simulink model "iqrdrls_simulink"  (R2012b)
settings: Solver=FixedStepDiscrete  SolverMode=SingleTasking  StartTime=0.0  StopTime=2450  RelTol=1e-3
libraries: dspsigops x5
settings Model: MinMaxOverflowLogging=MinMaxAndOverflow  FPTRunName=NoOverride  Creator=andreas  LastModifiedBy=andreas
settings DataIOCC: InspectSignalLogs=on
settings OptimizationCC: InlineParams=on  SimCompilerOptimization=On
settings DebuggingCC: SignalRangeChecking=warning  ParameterDowncastMsg=warning  ParameterOverflowMsg=warning  StrictBusMsg=ErrorOnBusTreatedAsVector  LoggingUnavailableSignals=none
settings HardwareCC: ProdHWDeviceType=Generic->Unspecified (assume 32-bit Generic)  TargetBitPerLong=64  TargetBitPerPointer=64  TargetIntDivRoundTo=Zero  TargetEndianess=LittleEndian  TargetWordSize=64  TargetHWDeviceType=MATLAB Host  ProdEqTarget=off
settings ModelReferenceCC: EnableParallelModelReferenceBuilds=on

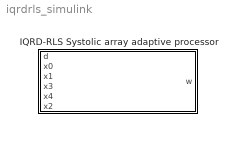
== system iqrdrls_simulink ==
  IQRD-RLS Systolic array adaptive processor : Subsystem

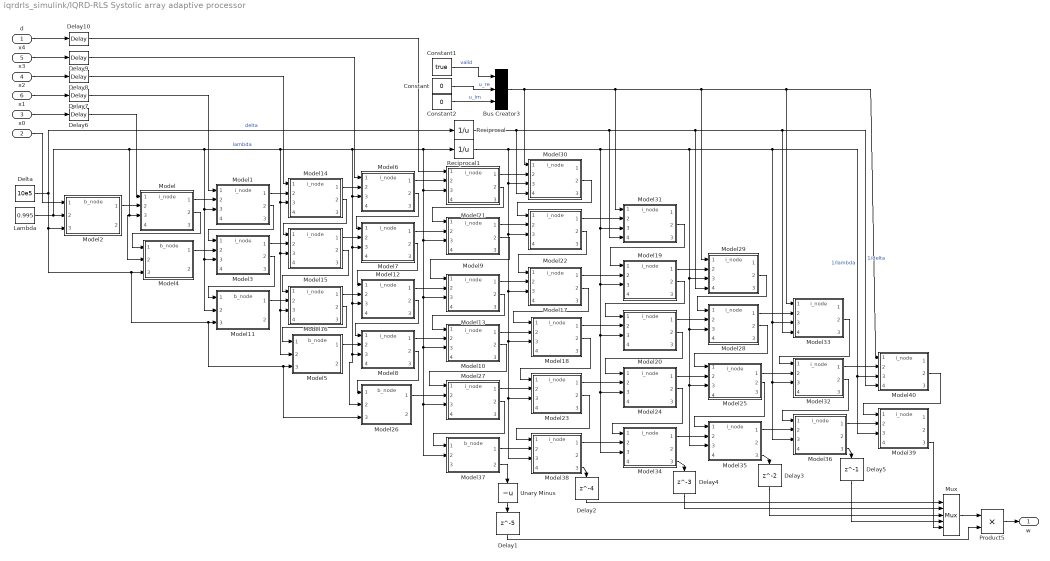
== system iqrdrls_simulink/IQRD-RLS Systolic array adaptive processor ==
  d : Inport  OutDataTypeStr=Bus: vbus
  x0 : Inport  Port=2  OutDataTypeStr=Bus: vbus
  x1 : Inport  Port=3  OutDataTypeStr=Bus: vbus
  x3 : Inport  Port=4  OutDataTypeStr=Bus: vbus
  x4 : Inport  Port=5  OutDataTypeStr=Bus: vbus
  x2 : Inport  Port=6  OutDataTypeStr=Bus: vbus
  Bus Creator3 : BusCreator  Inputs=3  OutDataTypeStr=Bus: vbus
  Constant : Constant  Value=0  VectorParams1D=off  OutDataTypeStr=double
  Constant1 : Constant  Value=true  OutDataTypeStr=boolean
  Constant2 : Constant  Value=0  VectorParams1D=off  OutDataTypeStr=double
  Delay1 : Delay  DelayLength=5  DelayLengthUpperLimit=20  InitialCondition=0
  Delay10 : dspsigops/Delay  InputProcessing=Columns as channels (frame based)  dly_unit=Samples  delay=5  ic_detail=off  dif_ic_for_ch=off  dif_ic_for_dly=off  ic=0  reset_popup=None
  Delay2 : Delay  DelayLength=4  DelayLengthUpperLimit=20  InitialCondition=0
  Delay3 : Delay  DelayLengthUpperLimit=20  InitialCondition=0
  Delay4 : Delay  DelayLength=3  DelayLengthUpperLimit=20  InitialCondition=0
  Delay5 : Delay  DelayLength=1  DelayLengthUpperLimit=20  InitialCondition=0
  Delay6 : dspsigops/Delay  InputProcessing=Columns as channels (frame based)  dly_unit=Samples  delay=1  ic_detail=off  dif_ic_for_ch=off  dif_ic_for_dly=off  ic=0  reset_popup=None
  Delay7 : dspsigops/Delay  InputProcessing=Columns as channels (frame based)  dly_unit=Samples  delay=2  ic_detail=off  dif_ic_for_ch=off  dif_ic_for_dly=off  ic=0  reset_popup=None
  Delay8 : dspsigops/Delay  InputProcessing=Columns as channels (frame based)  dly_unit=Samples  delay=3  ic_detail=off  dif_ic_for_ch=off  dif_ic_for_dly=off  ic=0  reset_popup=None
  Delay9 : dspsigops/Delay  InputProcessing=Columns as channels (frame based)  dly_unit=Samples  delay=4  ic_detail=off  dif_ic_for_ch=off  dif_ic_for_dly=off  ic=0  reset_popup=None
  Delta : Constant  Value=10e5  VectorParams1D=off  OutDataTypeStr=double
  Lambda : Constant  Value=0.995  VectorParams1D=off  OutDataTypeStr=double
  Model{,1,3,6..10,12..25,27..36,38..40} (35 alike) : ModelReference  ModelNameDialog=i_node  SimulationMode=Normal  ModelReferenceVersion=1.134  CopyOfModelName=i_node  DefaultDataLogging=on
  Model{2,4..5,11,26,37} (6 alike) : ModelReference  ModelNameDialog=b_node  SimulationMode=Normal  ModelReferenceVersion=1.97  CopyOfModelName=b_node  DefaultDataLogging=on
  Mux : Mux  Inputs=5
  Product5 : Product  OutDataTypeStr=double  RndMeth=Zero
  Reciprocal : Math  Operator=reciprocal  OutDataTypeStr=double  SaturateOnIntegerOverflow=on
  Reciprocal1 : Math  Operator=reciprocal  OutDataTypeStr=double  SaturateOnIntegerOverflow=on
  Unary Minus : UnaryMinus
  w : Outport
  wires:
  Constant/1 -> Bus Creator3/2  "u_re"
  Mux/1 -> Product5/1
  Model/1 -> Model1/2
  Model1/2 -> Model3/1
  Model2/1 -> Model/2
  Model/2 -> Model4/1
  Model4/1 -> Model3/2
  Model6/2 -> Model7/1
  Model7/1 -> Model9/2
  Model8/1 -> Model10/2
  Model5/1 -> Model8/2
  x0/1 -> Model2/1
  x1/1 -> Delay6/1
  d/1 -> Delay10/1
  Bus Creator3/1 -> Model29/1, Model33/1, Model40/1, Model31/1, Model30/1
  Constant1/1 -> Bus Creator3/1  "valid"
  Unary Minus/1 -> Delay1/1
  Delay2/1 -> Mux/1
  Delay4/1 -> Mux/2
  Model3/2 -> Model11/1
  Model7/2 -> Model12/1
  Model12/1 -> Model13/2
  Model12/2 -> Model8/1
  Model1/1 -> Model14/2
  Model14/2 -> Model15/1
  Model14/1 -> Model6/2
  Model15/1 -> Model7/2
  Model3/1 -> Model15/2
  Model15/2 -> Model16/1
  Model11/1 -> Model16/2
  Model16/1 -> Model12/2
  Model16/2 -> Model5/1
  Model13/2 -> Model10/1
  Model9/2 -> Model13/1
  Model13/1 -> Model17/2
  Model10/1 -> Model18/2
  Model17/2 -> Model18/1
  Delay3/1 -> Mux/3
  x2/1 -> Delay7/1
  Model8/2 -> Model26/1
  Model26/1 -> Model27/2
  Model27/1 -> Model23/2
  Model23/1 -> Model24/2
  Model10/2 -> Model27/1
  Model18/2 -> Model23/1
  Model20/2 -> Model24/1
  Model18/1 -> Model20/2
  Model17/1 -> Model19/2
  Model9/1 -> Model22/2
  Model22/2 -> Model17/1
  Model19/2 -> Model20/1
  Model24/1 -> Model25/2
  Lambda/1 -> Reciprocal1/1, Model37/2, Model27/3, Model10/3, Model13/3, Model9/3, Model21/3, Model26/2, Model8/3, Model12/3, Model7/3, Model6/3, Model5/2, Model16/3, Model15/3, Model14/3, Model11/2, Model3/3, Model1/3, Model4/2, Model/3, Model2/2  "lambda"
  Delta/1 -> Model2/3, Model26/3, Model5/3, Model11/3, Model4/3, Reciprocal/1  "delta"
  Model20/1 -> Model28/2
  Model28/2 -> Model25/1
  Delay1/1 -> Product5/2
  Model6/1 -> Model21/2
  Model21/2 -> Model9/1
  Model21/1 -> Model30/2
  Model22/1 -> Model31/2
  Model19/1 -> Model29/2
  Model28/1 -> Model33/2
  Model25/1 -> Model32/2
  Model30/2 -> Model22/1
  Model31/2 -> Model19/1
  Model29/2 -> Model28/1
  Model33/2 -> Model32/1
  Reciprocal1/1 -> Model30/3, Model38/3, Model23/3, Model18/3, Model17/3, Model22/3, Model40/3, Model39/3, Model33/3, Model32/3, Model36/3, Model29/3, Model28/3, Model25/3, Model35/3, Model31/3, Model19/3, Model20/3, Model24/3, Model34/3  "1/lambda"
  Model27/2 -> Model37/1
  Model23/2 -> Model38/1
  Model24/2 -> Model34/1
  Model25/2 -> Model35/1
  Model32/2 -> Model36/1
  Model40/2 -> Model39/1
  Model37/1 -> Model38/2
  Model38/1 -> Model34/2
  Model34/1 -> Model35/2
  Model35/1 -> Model36/2
  Model36/1 -> Model39/2
  Model32/1 -> Model40/2
  Reciprocal/1 -> Model30/4, Model40/4, Model33/4, Model29/4, Model31/4  "1/delta"
  x4/1 -> Delay9/1
  Model37/2 -> Unary Minus/1
  Model38/3 -> Delay2/1
  Model34/3 -> Delay4/1
  Model35/3 -> Delay3/1
  Model36/3 -> Delay5/1
  Model39/3 -> Mux/5
  Delay5/1 -> Mux/4
  Constant2/1 -> Bus Creator3/3  "u_im"
  x3/1 -> Delay8/1
  Product5/1 -> w/1
  Delay6/1 -> Model/1
  Delay7/1 -> Model1/1
  Delay8/1 -> Model14/1
  Delay9/1 -> Model6/1
  Delay10/1 -> Model21/1
